simulink model "ImpedenceControl"  (R2023a)
settings: Solver=FixedStepAuto  StartTime=0.0  StopTime=app.StopTime  FixedStep=.01  MaxStep=.1  RelTol=1e-5
undefined symbols (not defined in the file or in its folder): app, forwardKinematics, Generate_B, GenerateAnlyticalJacobian, TrimUnusedDofs_rows
settings Model: Creator=Ericw  LastModifiedBy=Ericw

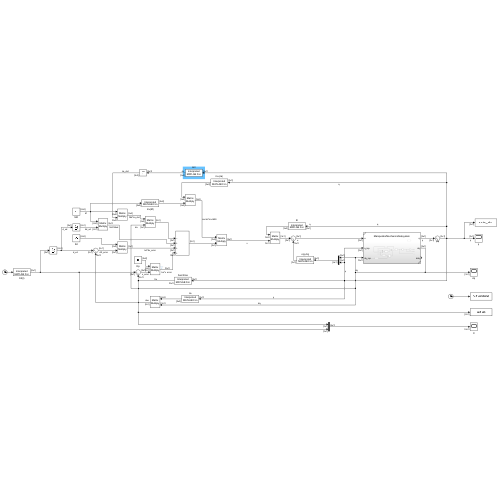
[thumbnail: Simulink's stored preview of the top-level diagram]
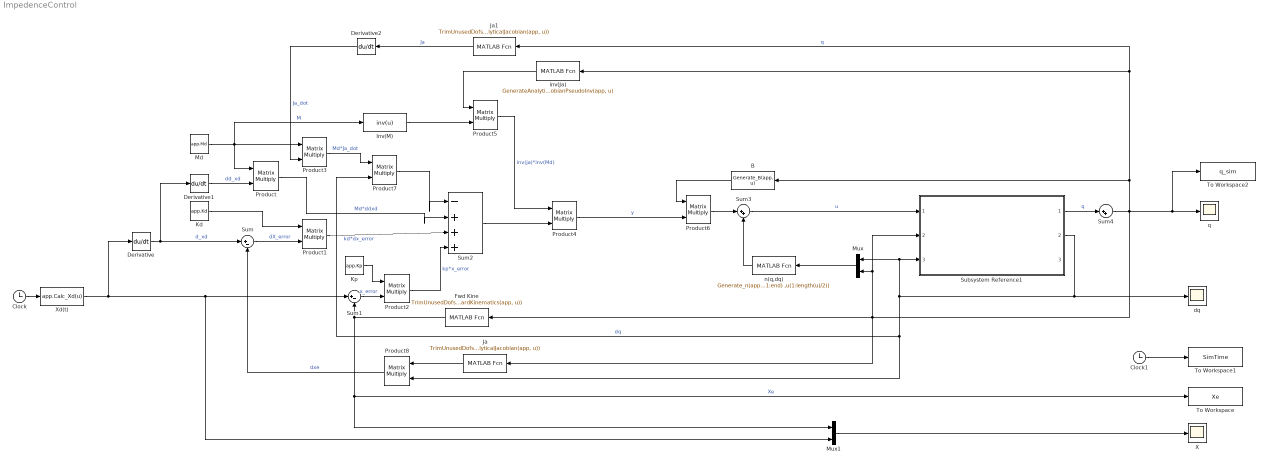
== system ImpedenceControl ==
  B : MATLABFcn  MATLABFcn=Generate_B(app, u)  OutputDimensions=[app.NumJoints,app.NumJoints]  Output1D=off
  Clock : Clock
  Clock1 : Clock
  Derivative : Derivative
  Derivative1 : Derivative
  Derivative2 : Derivative
  Fwd Kine : MATLABFcn  MATLABFcn=TrimUnusedDofs_rows(app,forwardKinematics(app, u))  OutputDimensions=[app.numActiveDofs,1]  Output1D=off
  Inv(M) : MATLABFcn  MATLABFcn=inv(u)  Output1D=off
  Ja : MATLABFcn  MATLABFcn=TrimUnusedDofs_rows(app,GenerateAnlyticalJacobian(app, u))  OutputDimensions=[app.numActiveDofs,app.NumJoints]  Output1D=off
  Ja1 : MATLABFcn  MATLABFcn=TrimUnusedDofs_rows(app,GenerateAnlyticalJacobian(app, u))  OutputDimensions=[app.numActiveDofs,app.NumJoints]  Output1D=off
  Kd : Constant  Value=app.Kd  VectorParams1D=off
  Kp : Constant  Value=app.Kp  VectorParams1D=off
  Md : Constant  Value=app.Md  VectorParams1D=off
  Mux : Mux  Inputs=2
  Mux1 : Mux  Inputs=2
  Product{,1..8} (9 alike) : Product  Multiplication=Matrix(*)
  Subsystem Reference1 : Subsystem  ReferencedSubsystem=ManipulatorMechanicsSubsystem
  Sum : Sum  Inputs=|+-
  Sum1 : Sum  Inputs=|+-
  Sum2 : Sum  Inputs=|-+++
  Sum3 : Sum  Inputs=|++
  Sum4 : Sum  Inputs=|++
  To Workspace : ToWorkspace  VariableName=Xe  SaveFormat=Timeseries  SampleTime=-1
  To Workspace1 : ToWorkspace  VariableName=SimTime  SaveFormat=Timeseries  SampleTime=-1
  To Workspace2 : ToWorkspace  VariableName=q_sim  SaveFormat=Timeseries  SampleTime=-1
  X : Scope
  Xd(t) : MATLABFcn  MATLABFcn=app.Calc_Xd(u)  OutputDimensions=[app.numActiveDofs,1]  Output1D=off
  dq : Scope
  inv(Ja) : MATLABFcn  MATLABFcn=GenerateAnalyticalJacobianPseudoInv(app, u)  Output1D=off
  n(q,dq) : MATLABFcn  MATLABFcn=Generate_n(app,u(length(u)/2+1:end) ,u(1:length(u)/2))  OutputDimensions=[app.NumJoints,1]  Output1D=off
  q : Scope
  wires:
  Derivative/1 -> Sum/1, Derivative1/1  "d_xd"
  Xd(t)/1 -> Mux1/2, Sum1/1, Derivative/1
  Product/1 -> Sum2/2  "Md*ddxd"
  Product1/1 -> Sum2/3  "kd*dx_error"
  Product2/1 -> Sum2/4  "kp*x_error"
  Kp/1 -> Product2/1
  Sum1/1 -> Product2/2  "x_error"
  Sum/1 -> Product1/2  "dX_error"
  Derivative1/1 -> Product/2  "dd_xd"
  Md/1 -> Product3/1, Inv(M)/1, Product/1  "M"
  Kd/1 -> Product1/1
  Sum2/1 -> Product4/2
  Product5/1 -> Product4/1  "inv(ja)*inv(Md)"
  Inv(M)/1 -> Product5/2
  inv(Ja)/1 -> Product5/1
  Product4/1 -> Product6/2  "y"
  B/1 -> Product6/1
  Product6/1 -> Sum3/1
  n(q,dq)/1 -> Sum3/2
  Product7/1 -> Sum2/1
  Sum4/1 -> To Workspace2/1, q/1, B/1, inv(Ja)/1, Ja1/1, Ja/1, Subsystem Reference1/2, Mux/2, Fwd Kine/1  "q"
  Subsystem Reference1/2 -> Mux/1, Subsystem Reference1/3, Product8/2, Product7/2, dq/1  "dq"
  Fwd Kine/1 -> Mux1/1, To Workspace/1, Sum1/2  "Xe"
  Ja/1 -> Product8/1
  Product8/1 -> Sum/2  "dxe"
  Product3/1 -> Product7/1  "Md*Ja_dot"
  Mux/1 -> n(q,dq)/1
  Clock/1 -> Xd(t)/1
  Clock1/1 -> To Workspace1/1
  Ja1/1 -> Derivative2/1  "Ja"
  Derivative2/1 -> Product3/2  "Ja_dot"
  Mux1/1 -> X/1
  Subsystem Reference1/1 -> Sum4/1  "q"
  Sum3/1 -> Subsystem Reference1/1  "u"
